simulink model "first_order_process"  (R2013a)
settings: Solver=ode45  StartTime=0  StopTime=1  RelTol=1e-3
values from neighbouring files (symbols this model uses):
  SAMPLING_INTERVAL = 10    [main_code.m]    (also in main_using_Torsche.m)
  StartTime = task{subtask_num}.start_time    [main_code.m]    (also in main_using_Torsche.m = task(subtask_num).start_time)
  x_initial_product_setpoint = last_setpoint    [main_code.m]    (also in main_using_Torsche.m)
  x_new_product_setpoint = task{subtask_num}.set_point    [main_code.m]    (also in main_using_Torsche.m = task(subtask_num).set_point)
  x_product_id = task{subtask_num}.product_id    [main_code.m]    (also in main_using_Torsche.m = task(subtask_num).product_id)
  x_throughput_setpoint = task{subtask_num}.speed    [main_code.m]    (also in main_using_Torsche.m = task(subtask_num).speed)
libraries: simulink x1
settings Model: Creator=acer  LastModifiedBy=acer
settings OptimizationCC: SimCompilerOptimization=On
settings HardwareCC: ProdBitPerInt=16  ProdBitPerPointer=8  ProdIntDivRoundTo=Zero  ProdWordSize=8  ProdShiftRightIntArith=off  ProdHWDeviceType=Intel->8051 Compatible
settings RTWCC: RTWCompilerOptimization=On

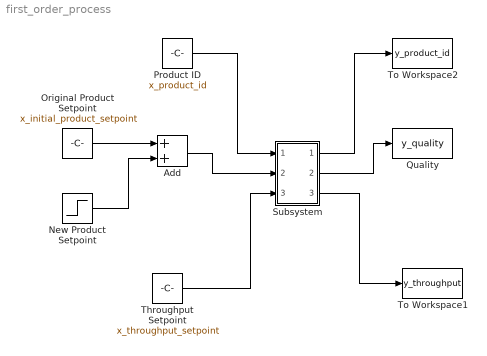
== system first_order_process ==
  Add : Sum
  New Product Setpoint : Step  Time=StartTime  After=x_new_product_setpoint - x_initial_product_setpoint  SampleTime=0
  Original Product Setpoint : Constant  Value=x_initial_product_setpoint
  Product ID : Constant  Value=x_product_id
  Quality : ToWorkspace  VariableName=y_quality  SampleTime=SAMPLING_INTERVAL  SaveFormat=Timeseries
  Subsystem : Subsystem
  Throughput Setpoint : Constant  Value=x_throughput_setpoint
  To Workspace1 : ToWorkspace  VariableName=y_throughput  SampleTime=SAMPLING_INTERVAL  SaveFormat=Timeseries
  To Workspace2 : ToWorkspace  VariableName=y_product_id  SampleTime=SAMPLING_INTERVAL  SaveFormat=Timeseries
  wires:
  Product ID/1 -> Subsystem/1(In1)
  Throughput Setpoint/1 -> Subsystem/3(In3)
  Subsystem/1(Out1) -> To Workspace2/1
  Subsystem/2(Out2) -> Quality/1
  Subsystem/3(Out3) -> To Workspace1/1
  Original Product Setpoint/1 -> Add/1
  New Product Setpoint/1 -> Add/2
  Add/1 -> Subsystem/2(In2)

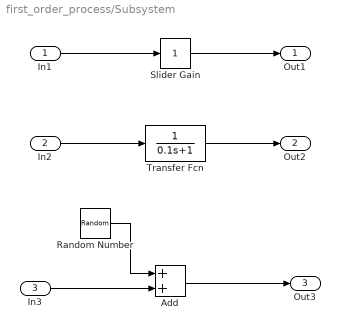
== system first_order_process/Subsystem ==
  In1 : Inport
  In2 : Inport  Port=2
  In3 : Inport  Port=3
  Add : Sum
  Random Number : RandomNumber  SampleTime=0
  Slider Gain : simulink/Math Operations/Slider Gain  low=0  gain=1  high=2
  Transfer Fcn : TransferFcn  Denominator=[0.1 1]
  Out1 : Outport
  Out2 : Outport  Port=2
  Out3 : Outport  Port=3
  wires:
  Slider Gain/1 -> Out1/1
  Transfer Fcn/1 -> Out2/1
  Random Number/1 -> Add/1
  Add/1 -> Out3/1
  In1/1 -> Slider Gain/1
  In2/1 -> Transfer Fcn/1
  In3/1 -> Add/2
